simulink model "simpleVehicleModel_forpp"  (R2017b)
settings: Solver=FixedStepAuto  StartTime=0.0  StopTime=0.22  FixedStep=0.01  RelTol=1e-3
values from neighbouring files (symbols this model uses):
  beta = x(i,j)    [pp_from_simple_model.m]
  delta = 0*pi/180    (= 0)    [pp_from_simple_model.m]
  g = 9.81    [initialize_simplemodel.m]    (also in initialize_simplemodel_Trial.m; tire_friction_circle.m)
  h = 0.35    [initialize_simplemodel.m]    (also in initialize_simplemodel_Trial.m)
  Izz = 1800    [initialize_simplemodel.m]    (also in initialize_simplemodel_Trial.m = 1400)
  lf = 1.4    [initialize_simplemodel.m]    (also in initialize_simplemodel_Trial.m)
  lr = 1.345    [initialize_simplemodel.m]    (also in initialize_simplemodel_Trial.m)
  m = 1400    [initialize_simplemodel.m]    (also in initialize_simplemodel_Trial.m = 1300; tire_friction_circle.m = 1300)
  r = 0.34    [initialize_simplemodel.m]    (also in initialize_simplemodel_Trial.m)
  steering_Gain = 12    [initialize_simplemodel.m]    (also in initialize_simplemodel_Trial.m)
  tr = 1.684/2    (= 0.842)    [initialize_simplemodel.m]    (also in initialize_simplemodel_Trial.m)
  vx = 10    [initialize_simplemodel_Trial.m]    (also in pp_from_simple_model.m; tire_friction_circle.m = 5)
undefined symbols (not defined in the file or in its folder): DiscIntNeverNeededParam, psi_dot
libraries: simulink x1
settings Model: Creator=ashwin.ramanujam  LastModifiedBy=gandh

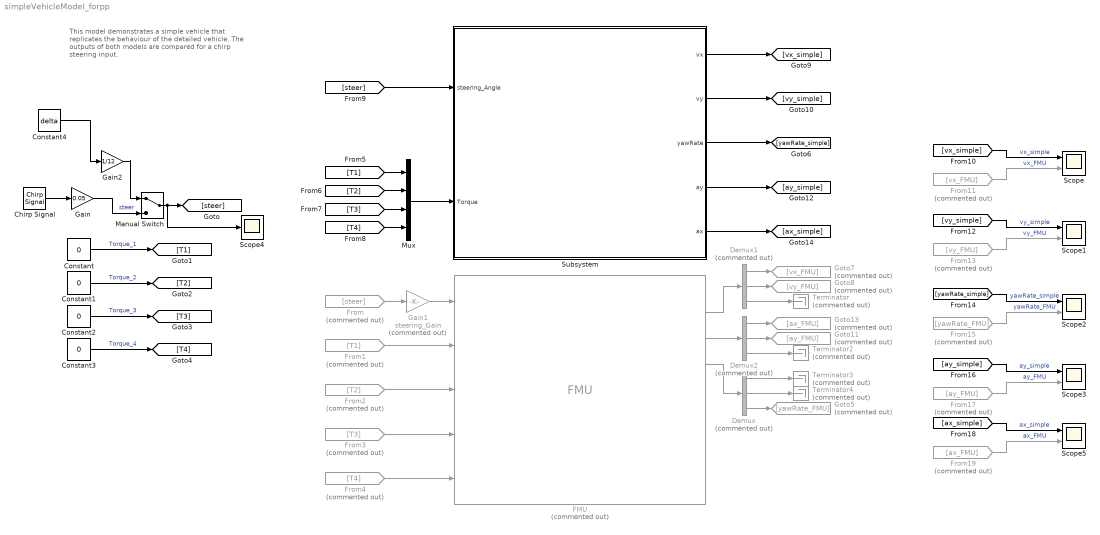
== system simpleVehicleModel_forpp ==
  note: This model demonstrates a simple vehicle that replicates the behaviour of the detailed vehicle. The outputs of both models are compared for a chirp steering input.
  Chirp Signal : simulink/Sources/Chirp Signal  f1=1  T=10  f2=4
  Constant{,1..3} (4 alike) : Constant  Value=0
  Constant4 : Constant  Value=delta
  Demux : Demux  Commented=on  Outputs=3
  Demux1 : Demux  Commented=on  Outputs=3
  Demux2 : Demux  Commented=on  Outputs=3
  FMU : FMU  Commented=on  FMUName=MED2018_VehicleModel.fmu  FMUMode=CoSimulation  FMUSampleTime=-1  mask(MED2018.VehicleModel [Co-Simulation, v2.0]){}
  From : From  Commented=on  GotoTag=steer
  From1 : From  Commented=on  GotoTag=T1
  From11 : From  Commented=on  GotoTag=vx_FMU
  From13 : From  Commented=on  GotoTag=vy_FMU
  From15 : From  Commented=on  GotoTag=yawRate_FMU
  From17 : From  Commented=on  GotoTag=ay_FMU
  From19 : From  Commented=on  GotoTag=ax_FMU
  From2 : From  Commented=on  GotoTag=T2
  From3 : From  Commented=on  GotoTag=T3
  From4 : From  Commented=on  GotoTag=T4
  Gain : Gain  Gain=0.05
  Gain1 : Gain  Commented=on  Gain=steering_Gain
  Gain2 : Gain  Gain=1/12
  Goto11 : Goto  Commented=on  GotoTag=ay_FMU
  Goto13 : Goto  Commented=on  GotoTag=ax_FMU
  Goto5 : Goto  Commented=on  GotoTag=yawRate_FMU
  Goto7 : Goto  Commented=on  GotoTag=vx_FMU
  Goto8 : Goto  Commented=on  GotoTag=vy_FMU
  Manual Switch : ManualSwitch
  Mux : Mux
  Scope{,1..3,5} (5 alike) : Scope  NumInputPorts=2
  Scope4 : Scope
  Subsystem : Subsystem
  Terminator{,2..4} (4 alike) : Terminator  Commented=on
  wires:
  Mux/1 -> Subsystem/2(Torque)
  FMU/4 -> Demux/1
  Demux/3 -> Goto5/1
  Gain1/1 -> FMU/1
  Chirp Signal/1 -> Gain/1
  Constant/1 -> [T1]  "Torque_1"
  Constant1/1 -> [T2]  "Torque_2"
  Constant2/1 -> [T3]  "Torque_3"
  Constant3/1 -> [T4]  "Torque_4"
  From/1 -> Gain1/1
  From4/1 -> FMU/5
  From1/1 -> FMU/2
  From2/1 -> FMU/3
  From3/1 -> FMU/4
  [T1] -> Mux/1
  [T2] -> Mux/2
  [T3] -> Mux/3
  [T4] -> Mux/4
  Subsystem/3(yawRate) -> [yawRate_simple]
  FMU/2 -> Demux1/1
  Demux1/1 -> Goto7/1
  Demux1/2 -> Goto8/1
  Subsystem/1(vx) -> [vx_simple]
  Subsystem/2(vy) -> [vy_simple]
  [vx_simple] -> Scope/1  "vx_simple"
  From11/1 -> Scope/2  "vx_FMU"
  From13/1 -> Scope1/2  "vy_FMU"
  [vy_simple] -> Scope1/1  "vy_simple"
  From15/1 -> Scope2/2  "yawRate_FMU"
  [yawRate_simple] -> Scope2/1  "yawRate_simple"
  Gain/1 -> Manual Switch/2  "steer"
  [steer] -> Subsystem/1(steering_Angle)
  FMU/3 -> Demux2/1
  Demux2/2 -> Goto11/1
  Subsystem/4(ay) -> [ay_simple]
  From17/1 -> Scope3/2  "ay_FMU"
  [ay_simple] -> Scope3/1  "ay_simple"
  Demux1/3 -> Terminator/1
  Demux2/1 -> Goto13/1
  Demux2/3 -> Terminator2/1
  Demux/1 -> Terminator3/1
  Demux/2 -> Terminator4/1
  Subsystem/5(ax) -> [ax_simple]
  [ax_simple] -> Scope5/1  "ax_simple"
  From19/1 -> Scope5/2  "ax_FMU"
  Constant4/1 -> Gain2/1
  Manual Switch/1 -> Scope4/1, [steer]
  Gain2/1 -> Manual Switch/1

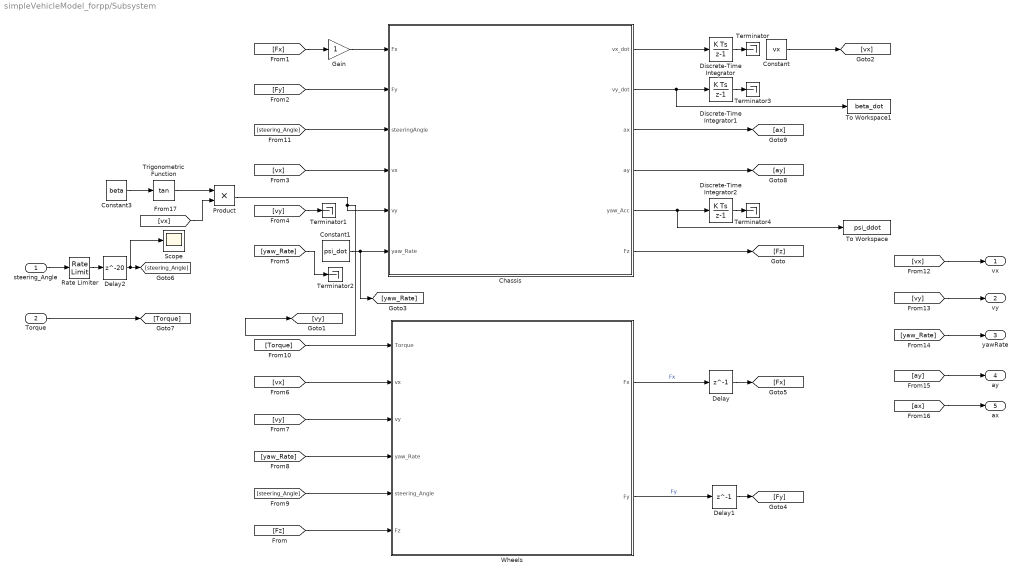
== system simpleVehicleModel_forpp/Subsystem ==
  steering_Angle : Inport
  Torque : Inport  Port=2
  Chassis : MATLAB Function  TreatAsAtomicUnit=on
  Constant : Constant  Value=vx
  Constant1 : Constant  Value=psi_dot
  Constant3 : Constant  Value=beta
  Delay : Delay  DelayLength=1  InitialCondition=[m*g*lr/(lf+lr)/2;m*g*lr/(lf+lr)/2;m*g*lf/(lf+lr)/2;m*g*lf/(lf+lr)/2]
  Delay1 : Delay  DelayLength=1  InitialCondition=[m*g*lr/(lf+lr)/2;m*g*lr/(lf+lr)/2;m*g*lf/(lf+lr)/2;m*g*lf/(lf+lr)/2]
  Delay2 : Delay  DelayLength=20  InitialCondition=0
  Discrete-Time Integrator : DiscreteIntegrator  InitialCondition=60*5/18  InitialConditionSetting=State (most efficient)  SampleTime=-1  ICPrevOutput=DiscIntNeverNeededParam  ICPrevScaledInput=DiscIntNeverNeededParam
  Discrete-Time Integrator1 : DiscreteIntegrator  InitialConditionSetting=State (most efficient)  SampleTime=-1  ICPrevOutput=DiscIntNeverNeededParam  ICPrevScaledInput=DiscIntNeverNeededParam
  Discrete-Time Integrator2 : DiscreteIntegrator  InitialConditionSetting=State (most efficient)  SampleTime=-1  ICPrevOutput=DiscIntNeverNeededParam  ICPrevScaledInput=DiscIntNeverNeededParam
  Gain : Gain
  Product : Product
  Rate Limiter : RateLimiter  RisingSlewLimit=500*pi/180/12  FallingSlewLimit=-500*pi/180/12  SampleTimeMode=inherited
  Scope : Scope
  Terminator{,1..4} (5 alike) : Terminator
  To Workspace : ToWorkspace  VariableName=psi_ddot  SaveFormat=Timeseries  SampleTime=-1
  To Workspace1 : ToWorkspace  VariableName=beta_dot  SaveFormat=Timeseries  SampleTime=-1
  Trigonometric Function : Trigonometry  Operator=tan
  Wheels : Subsystem  Priority=0
  vx : Outport
  vy : Outport  Port=2
  yawRate : Outport  Port=3
  ay : Outport  Port=4
  ax : Outport  Port=5
  wires:
  [vx] -> Chassis/4(vx)
  Discrete-Time Integrator2/1 -> Terminator4/1
  [Fy] -> Chassis/2(Fy)
  [vy] -> Wheels/3(vy)
  [Torque] -> Wheels/1(Torque)
  [yaw_Rate] -> yawRate/1
  [yaw_Rate] -> Wheels/4(yaw_Rate)
  [vx] -> vx/1
  [vx] -> Wheels/2(vx)
  [Fz] -> Wheels/6(Fz)
  [steering_Angle] -> Chassis/3(steeringAngle)
  [steering_Angle] -> Wheels/5(steering_Angle)
  steering_Angle/1 -> Rate Limiter/1
  Torque/1 -> [Torque]
  [vy] -> vy/1
  Chassis/5(yaw_Acc) -> To Workspace/1, Discrete-Time Integrator2/1
  [Fx] -> Gain/1
  Wheels/1(Fx) -> Delay/1  "Fx"
  Wheels/2(Fy) -> Delay1/1  "Fy"
  Chassis/6(Fz) -> [Fz]
  Rate Limiter/1 -> Delay2/1
  Delay2/1 -> Scope/1, [steering_Angle]
  [ay] -> ay/1
  Delay/1 -> [Fx]
  Delay1/1 -> [Fy]
  Chassis/1(vx_dot) -> Discrete-Time Integrator/1
  Chassis/4(ay) -> [ay]
  Chassis/3(ax) -> [ax]
  [ax] -> ax/1
  Constant/1 -> [vx]
  Constant3/1 -> Trigonometric Function/1
  Trigonometric Function/1 -> Product/1
  Product/1 -> [vy], Chassis/5(vy)
  Constant1/1 -> [yaw_Rate], Chassis/6(yaw_Rate)
  [vx] -> Product/2
  Chassis/2(vy_dot) -> To Workspace1/1, Discrete-Time Integrator1/1
  Discrete-Time Integrator/1 -> Terminator/1
  [vy] -> Terminator1/1
  [yaw_Rate] -> Terminator2/1
  Gain/1 -> Chassis/1(Fx)
  Discrete-Time Integrator1/1 -> Terminator3/1

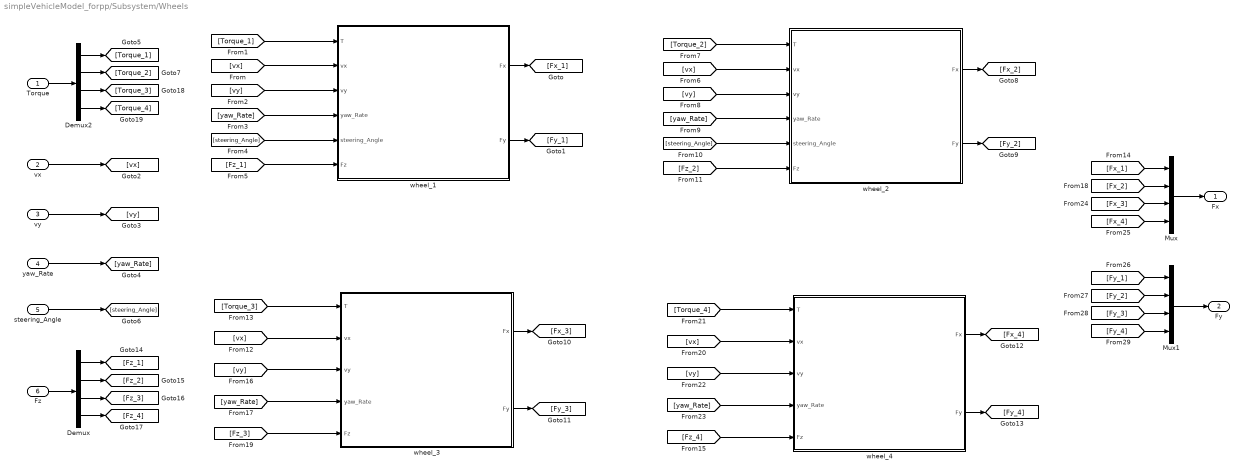
== system simpleVehicleModel_forpp/Subsystem/Wheels ==
  Torque : Inport
  vx : Inport  Port=2
  vy : Inport  Port=3
  yaw_Rate : Inport  Port=4
  steering_Angle : Inport  Port=5
  Fz : Inport  Port=6
  Demux : Demux
  Demux2 : Demux
  Mux : Mux
  Mux1 : Mux
  wheel_1 : Subsystem
  wheel_2 : Subsystem
  wheel_3 : Subsystem
  wheel_4 : Subsystem
  Fx : Outport
  Fy : Outport  Port=2
  wires:
  vx/1 -> [vx]
  vy/1 -> [vy]
  yaw_Rate/1 -> [yaw_Rate]
  [vx] -> wheel_1/2(vx)
  wheel_1/1(Fx) -> [Fx_1]
  wheel_1/2(Fy) -> [Fy_1]
  [steering_Angle] -> wheel_1/5(steering_Angle)
  [yaw_Rate] -> wheel_1/4(yaw_Rate)
  [vy] -> wheel_1/3(vy)
  [Torque_1] -> wheel_1/1(T)
  steering_Angle/1 -> [steering_Angle]
  wheel_2/1(Fx) -> [Fx_2]
  wheel_2/2(Fy) -> [Fy_2]
  [yaw_Rate] -> wheel_2/4(yaw_Rate)
  [vy] -> wheel_2/3(vy)
  [steering_Angle] -> wheel_2/5(steering_Angle)
  [vx] -> wheel_2/2(vx)
  wheel_3/1(Fx) -> [Fx_3]
  [yaw_Rate] -> wheel_3/4(yaw_Rate)
  [vy] -> wheel_4/3(vy)
  [yaw_Rate] -> wheel_4/4(yaw_Rate)
  [vx] -> wheel_4/2(vx)
  wheel_4/2(Fy) -> [Fy_4]
  wheel_3/2(Fy) -> [Fy_3]
  wheel_4/1(Fx) -> [Fx_4]
  [vy] -> wheel_3/3(vy)
  [vx] -> wheel_3/2(vx)
  [Fx_1] -> Mux/1
  [Fx_2] -> Mux/2
  [Fx_3] -> Mux/3
  [Fx_4] -> Mux/4
  [Fy_3] -> Mux1/3
  [Fy_4] -> Mux1/4
  [Fy_2] -> Mux1/2
  [Fy_1] -> Mux1/1
  Demux/1 -> [Fz_1]
  Demux/2 -> [Fz_2]
  Demux/3 -> [Fz_3]
  Demux/4 -> [Fz_4]
  [Fz_1] -> wheel_1/6(Fz)
  [Fz_3] -> wheel_3/5(Fz)
  [Fz_4] -> wheel_4/5(Fz)
  [Fz_2] -> wheel_2/6(Fz)
  Fz/1 -> Demux/1
  [Torque_3] -> wheel_3/1(T)
  [Torque_2] -> wheel_2/1(T)
  [Torque_4] -> wheel_4/1(T)
  Demux2/4 -> [Torque_4]
  Demux2/3 -> [Torque_3]
  Demux2/1 -> [Torque_1]
  Torque/1 -> Demux2/1
  Demux2/2 -> [Torque_2]
  Mux1/1 -> Fy/1
  Mux/1 -> Fx/1

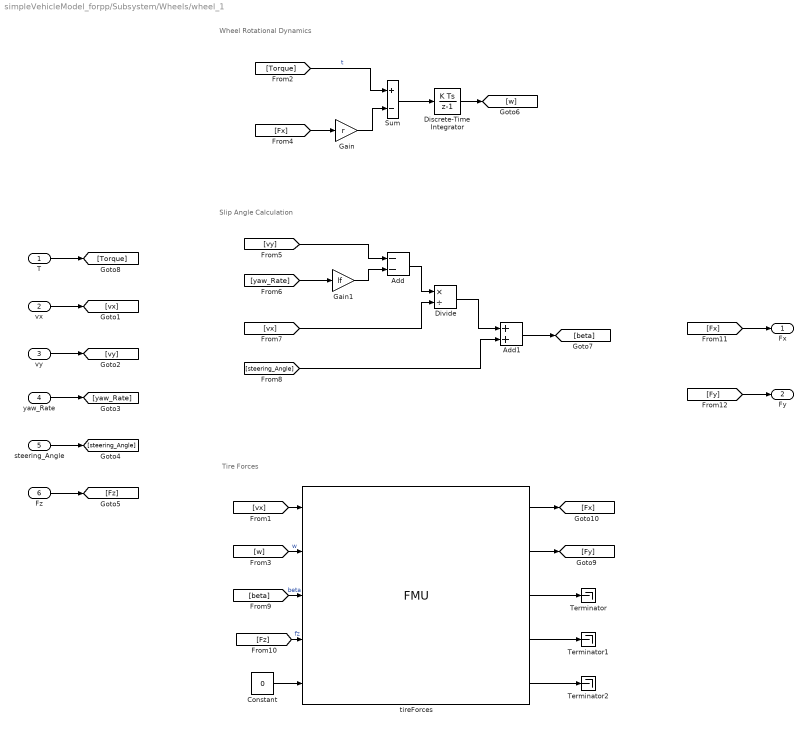
== system simpleVehicleModel_forpp/Subsystem/Wheels/wheel_1 ==
  note: Tire Forces
  note: Wheel Rotational Dynamics
  note: Slip Angle Calculation
  T : Inport
  vx : Inport  Port=2
  vy : Inport  Port=3
  yaw_Rate : Inport  Port=4
  steering_Angle : Inport  Port=5
  Fz : Inport  Port=6
  Add : Sum  Inputs=--
  Add1 : Sum
  Constant : Constant  Value=0
  Discrete-Time Integrator : DiscreteIntegrator  InitialConditionSetting=State (most efficient)  SampleTime=-1  ICPrevOutput=DiscIntNeverNeededParam  ICPrevScaledInput=DiscIntNeverNeededParam
  Divide : Product  Inputs=*/
  Gain : Gain  Gain=r
  Gain1 : Gain  Gain=lf
  Sum : Sum  Inputs=+-
  Terminator : Terminator
  Terminator1 : Terminator
  Terminator2 : Terminator
  tireForces : FMU  FMUName=MED2018_TireModel.fmu  FMUMode=CoSimulation  FMUSampleTime=-1  mask(TyreFMUContainer [Co-Simulation, v2.0]){}
  Fx : Outport
  Fy : Outport  Port=2
  wires:
  Discrete-Time Integrator/1 -> [w]
  tireForces/5 -> Terminator2/1
  tireForces/2 -> [Fy]
  tireForces/4 -> Terminator1/1
  tireForces/3 -> Terminator/1
  Sum/1 -> Discrete-Time Integrator/1
  [Torque] -> Sum/1  "t"
  Gain/1 -> Sum/2
  [Fx] -> Gain/1
  Constant/1 -> tireForces/5
  Gain1/1 -> Add/2
  Add/1 -> Divide/1
  [w] -> tireForces/2  "w"
  vx/1 -> [vx]
  vy/1 -> [vy]
  steering_Angle/1 -> [steering_Angle]
  yaw_Rate/1 -> [yaw_Rate]
  Fz/1 -> [Fz]
  [vx] -> tireForces/1
  [vy] -> Add/1
  [yaw_Rate] -> Gain1/1
  [vx] -> Divide/2
  Divide/1 -> Add1/1
  [steering_Angle] -> Add1/2
  Add1/1 -> [beta]
  [beta] -> tireForces/3  "beta"
  [Fz] -> tireForces/4  "fz"
  T/1 -> [Torque]
  tireForces/1 -> [Fx]
  [Fx] -> Fx/1
  [Fy] -> Fy/1

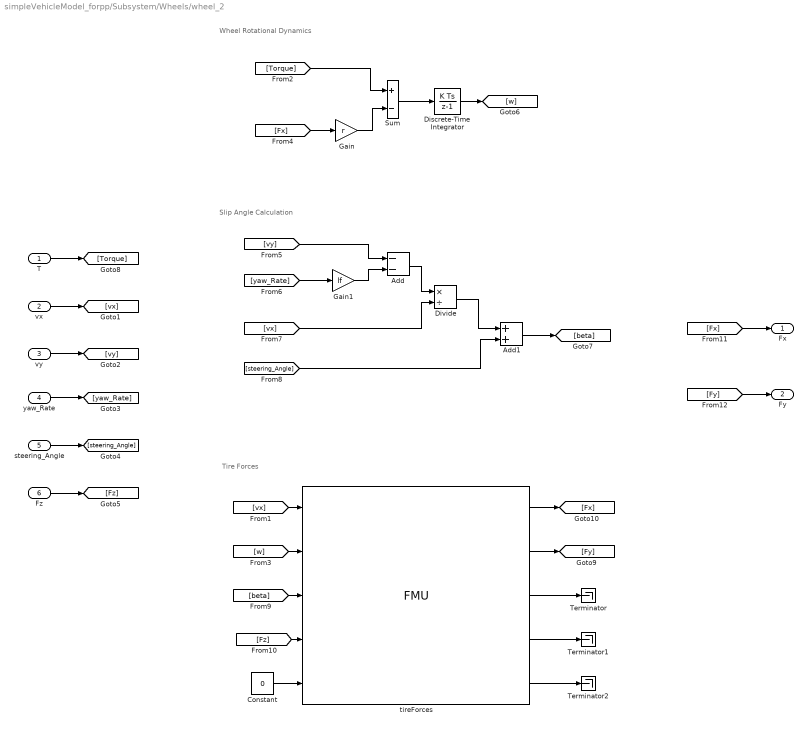
== system simpleVehicleModel_forpp/Subsystem/Wheels/wheel_2 ==
  note: Tire Forces
  note: Wheel Rotational Dynamics
  note: Slip Angle Calculation
  T : Inport
  vx : Inport  Port=2
  vy : Inport  Port=3
  yaw_Rate : Inport  Port=4
  steering_Angle : Inport  Port=5
  Fz : Inport  Port=6
  Add : Sum  Inputs=--
  Add1 : Sum
  Constant : Constant  Value=0
  Discrete-Time Integrator : DiscreteIntegrator  InitialConditionSetting=State (most efficient)  SampleTime=-1  ICPrevOutput=DiscIntNeverNeededParam  ICPrevScaledInput=DiscIntNeverNeededParam
  Divide : Product  Inputs=*/
  Gain : Gain  Gain=r
  Gain1 : Gain  Gain=lf
  Sum : Sum  Inputs=+-
  Terminator : Terminator
  Terminator1 : Terminator
  Terminator2 : Terminator
  tireForces : FMU  FMUName=MED2018_TireModel.fmu  FMUMode=CoSimulation  FMUSampleTime=-1  mask(TyreFMUContainer [Co-Simulation, v2.0]){}
  Fx : Outport
  Fy : Outport  Port=2
  wires:
  Discrete-Time Integrator/1 -> [w]
  tireForces/5 -> Terminator2/1
  tireForces/2 -> [Fy]
  tireForces/4 -> Terminator1/1
  tireForces/3 -> Terminator/1
  Sum/1 -> Discrete-Time Integrator/1
  [Torque] -> Sum/1
  Gain/1 -> Sum/2
  [Fx] -> Gain/1
  Constant/1 -> tireForces/5
  Gain1/1 -> Add/2
  Add/1 -> Divide/1
  [w] -> tireForces/2
  vx/1 -> [vx]
  vy/1 -> [vy]
  steering_Angle/1 -> [steering_Angle]
  yaw_Rate/1 -> [yaw_Rate]
  Fz/1 -> [Fz]
  [vx] -> tireForces/1
  [vy] -> Add/1
  [yaw_Rate] -> Gain1/1
  [vx] -> Divide/2
  Divide/1 -> Add1/1
  [steering_Angle] -> Add1/2
  Add1/1 -> [beta]
  [beta] -> tireForces/3
  [Fz] -> tireForces/4
  T/1 -> [Torque]
  tireForces/1 -> [Fx]
  [Fx] -> Fx/1
  [Fy] -> Fy/1

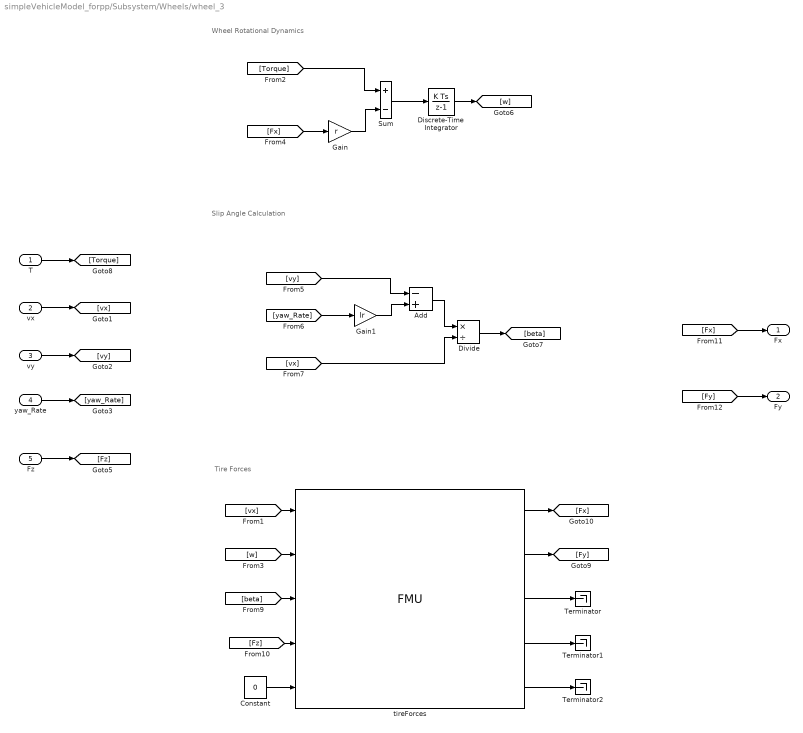
== system simpleVehicleModel_forpp/Subsystem/Wheels/wheel_3 ==
  note: Tire Forces
  note: Wheel Rotational Dynamics
  note: Slip Angle Calculation
  T : Inport
  vx : Inport  Port=2
  vy : Inport  Port=3
  yaw_Rate : Inport  Port=4
  Fz : Inport  Port=5
  Add : Sum  Inputs=-+
  Constant : Constant  Value=0
  Discrete-Time Integrator : DiscreteIntegrator  InitialConditionSetting=State (most efficient)  SampleTime=-1  ICPrevOutput=DiscIntNeverNeededParam  ICPrevScaledInput=DiscIntNeverNeededParam
  Divide : Product  Inputs=*/
  Gain : Gain  Gain=r
  Gain1 : Gain  Gain=lr
  Sum : Sum  Inputs=+-
  Terminator : Terminator
  Terminator1 : Terminator
  Terminator2 : Terminator
  tireForces : FMU  FMUName=MED2018_TireModel.fmu  FMUMode=CoSimulation  FMUSampleTime=-1  mask(TyreFMUContainer [Co-Simulation, v2.0]){}
  Fx : Outport
  Fy : Outport  Port=2
  wires:
  Discrete-Time Integrator/1 -> [w]
  tireForces/5 -> Terminator2/1
  tireForces/2 -> [Fy]
  tireForces/4 -> Terminator1/1
  tireForces/3 -> Terminator/1
  Sum/1 -> Discrete-Time Integrator/1
  [Torque] -> Sum/1
  Gain/1 -> Sum/2
  [Fx] -> Gain/1
  Constant/1 -> tireForces/5
  Gain1/1 -> Add/2
  Add/1 -> Divide/1
  [w] -> tireForces/2
  vx/1 -> [vx]
  vy/1 -> [vy]
  yaw_Rate/1 -> [yaw_Rate]
  Fz/1 -> [Fz]
  [vx] -> tireForces/1
  [vy] -> Add/1
  [yaw_Rate] -> Gain1/1
  [vx] -> Divide/2
  [beta] -> tireForces/3
  [Fz] -> tireForces/4
  T/1 -> [Torque]
  tireForces/1 -> [Fx]
  [Fx] -> Fx/1
  [Fy] -> Fy/1
  Divide/1 -> [beta]

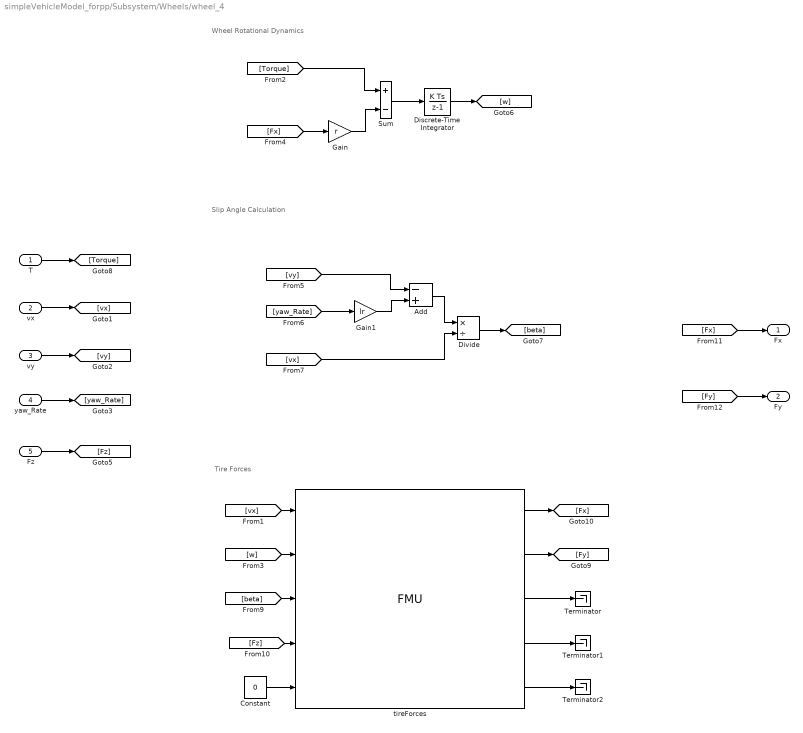
== system simpleVehicleModel_forpp/Subsystem/Wheels/wheel_4 ==
  note: Tire Forces
  note: Wheel Rotational Dynamics
  note: Slip Angle Calculation
  T : Inport
  vx : Inport  Port=2
  vy : Inport  Port=3
  yaw_Rate : Inport  Port=4
  Fz : Inport  Port=5
  Add : Sum  Inputs=-+
  Constant : Constant  Value=0
  Discrete-Time Integrator : DiscreteIntegrator  InitialConditionSetting=State (most efficient)  SampleTime=-1  ICPrevOutput=DiscIntNeverNeededParam  ICPrevScaledInput=DiscIntNeverNeededParam
  Divide : Product  Inputs=*/
  Gain : Gain  Gain=r
  Gain1 : Gain  Gain=lr
  Sum : Sum  Inputs=+-
  Terminator : Terminator
  Terminator1 : Terminator
  Terminator2 : Terminator
  tireForces : FMU  FMUName=MED2018_TireModel.fmu  FMUDebugLogging=on  FMUMode=CoSimulation  FMUSampleTime=-1  mask(TyreFMUContainer [Co-Simulation, v2.0]){}
  Fx : Outport
  Fy : Outport  Port=2
  wires:
  Discrete-Time Integrator/1 -> [w]
  tireForces/5 -> Terminator2/1
  tireForces/2 -> [Fy]
  tireForces/4 -> Terminator1/1
  tireForces/3 -> Terminator/1
  Sum/1 -> Discrete-Time Integrator/1
  [Torque] -> Sum/1
  Gain/1 -> Sum/2
  [Fx] -> Gain/1
  Constant/1 -> tireForces/5
  [w] -> tireForces/2
  vx/1 -> [vx]
  vy/1 -> [vy]
  yaw_Rate/1 -> [yaw_Rate]
  Fz/1 -> [Fz]
  [vx] -> tireForces/1
  [beta] -> tireForces/3
  [Fz] -> tireForces/4
  T/1 -> [Torque]
  tireForces/1 -> [Fx]
  [Fx] -> Fx/1
  [Fy] -> Fy/1
  [vy] -> Add/1
  [vx] -> Divide/2
  [yaw_Rate] -> Gain1/1
  Add/1 -> Divide/1
  Gain1/1 -> Add/2
  Divide/1 -> [beta]

== matlab function simpleVehicleModel_forpp/Subsystem/Chassis ==
  data: vx_dot output; vy_dot output; Fx input; Fy input; steeringAngle input; vx input; vy input; yaw_Rate input; ax output; ay output; yaw_Acc output; Fz output; g parameter; h parameter; Izz parameter; lf parameter; lr parameter; m parameter; tf parameter; tr parameter
function [vx_dot, vy_dot, ax, ay, yaw_Acc, Fz] = vehicleModel(Fx, Fy, steeringAngle, vx, vy, yaw_Rate, g, h, Izz, lf, lr, m, tf, tr)

% Function to simulate vehicle body
% Vehicle Parameters must be loaded from init.m

%Model Equations

fx = (Fx(1)+Fx(2))*cos(steeringAngle) - (Fy(1)+Fy(2))*sin(steeringAngle) + Fx(3) + Fx(4);
fy = (Fx(1)+Fx(2))*sin(steeringAngle) + (Fy(1)+Fy(2))*cos(steeringAngle) + Fy(3) + Fy(4);
Mz =  lf*((Fx(1)+Fx(2))*sin(steeringAngle) + (Fy(1)+Fy(2))*cos(steeringAngle))...
    + tf*((-Fx(1)+Fx(2))*cos(steeringAngle) + (Fy(1)-Fy(2))*sin(steeringAngle))...
    - lr*(Fy(3)+Fy(4)) + tr*(-Fx(3)+Fx(4));

ax = fx/m;
ay = fy/m;

vx_dot      = ax + vy*yaw_Rate;
vy_dot      = ay - vx*yaw_Rate;
yaw_Acc = Mz/Izz;

Fz = zeros(4,1);%[m*g*lr/(lf+lr)/2;m*g*lr/(lf+lr)/2;m*g*lf/(lf+lr)/2;m*g*lf/(lf+lr)/2];
Fz(1) = m * (g*lr/(lf+lr)/2 - ax*h/(lf+lr)/2 - ay*h/tf/2);
Fz(2) = m * (g*lr/(lf+lr)/2 - ax*h/(lf+lr)/2 + ay*h/tf/2);
Fz(3) = m * (g*lf/(lf+lr)/2 + ax*h/(lf+lr)/2 - ay*h/tr/2);
Fz(4) = m * (g*lf/(lf+lr)/2 + ax*h/(lf+lr)/2 + ay*h/tr/2);
